simulink model "intes_cross_2018b_0110_2"  (R2018b)
settings: Solver=VariableStepAuto  StartTime=0.0  StopTime=10.0  RelTol=1e-3
values from neighbouring files (symbols this model uses):
  k_ZOP_V2X_Enable = 1.0    [ZOP_Func.sldd]
settings Model: Creator=lenovo  LastModifiedBy=lenovo

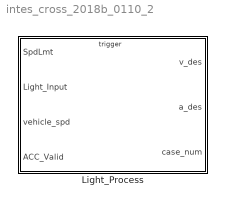
== system intes_cross_2018b_0110_2 ==
  Light_Process : Subsystem

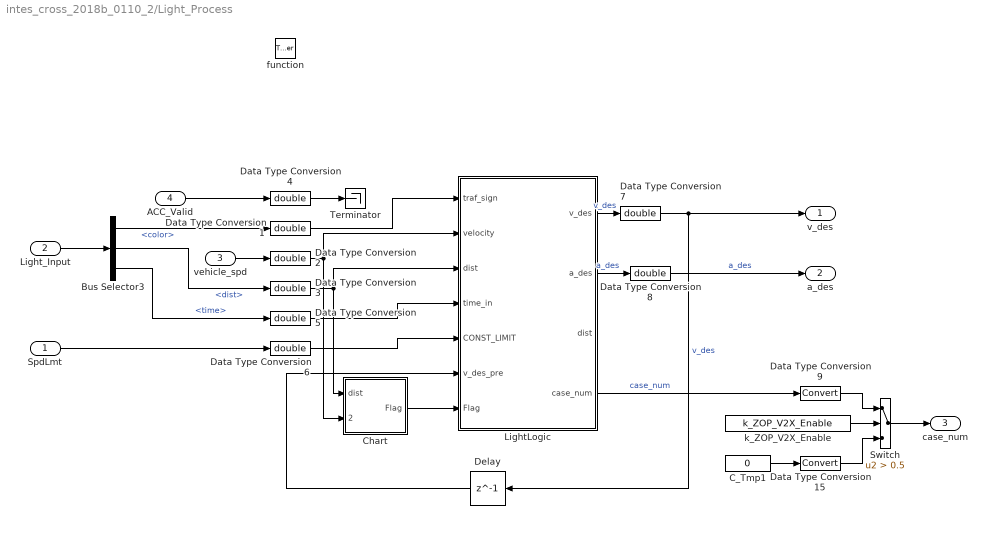
== system intes_cross_2018b_0110_2/Light_Process ==
  SpdLmt : Inport  BusOutputAsStruct=on
  Light_Input : Inport  Port=2  OutDataTypeStr=Bus: Light_Info_ST  BusOutputAsStruct=on
  vehicle_spd : Inport  Port=3  BusOutputAsStruct=on
  ACC_Valid : Inport  Port=4  BusOutputAsStruct=on
  function : TriggerPort  TriggerType=function-call  VariantControl=Variant
  Bus Selector3 : BusSelector  OutputSignals=color,dist,time
  C_Tmp1 : Constant  Value=0
  Chart : Stateflow chart  TreatAsAtomicUnit=on
  Data Type Conversion{1..8} (8 alike) : DataTypeConversion  OutDataTypeStr=double
  Data Type Conversion15 : DataTypeConversion
  Data Type Conversion9 : DataTypeConversion
  Delay : Delay  DelayLength=1
  LightLogic : MATLAB Function  TreatAsAtomicUnit=on
  Switch : Switch  Criteria=u2 > Threshold  Threshold=0.5
  Terminator : Terminator
  k_ZOP_V2X_Enable : Constant  Value=k_ZOP_V2X_Enable
  v_des : Outport
  a_des : Outport  Port=2
  case_num : Outport  Port=3
  wires:
  Data Type Conversion7/1 -> v_des/1, Delay/1  "v_des"
  Delay/1 -> LightLogic/6(v_des_pre)
  Light_Input/1 -> Bus Selector3/1
  ACC_Valid/1 -> Data Type Conversion4/1
  Data Type Conversion8/1 -> a_des/1  "a_des"
  Bus Selector3/1 -> Data Type Conversion1/1  "<color>"
  Bus Selector3/2 -> Data Type Conversion3/1  "<dist>"
  vehicle_spd/1 -> Data Type Conversion2/1
  Bus Selector3/3 -> Data Type Conversion5/1  "<time>"
  Data Type Conversion1/1 -> LightLogic/1(traf_sign)
  Data Type Conversion3/1 -> LightLogic/3("dist "), Chart/1(dist)
  Data Type Conversion5/1 -> LightLogic/4(time_in)
  Data Type Conversion6/1 -> LightLogic/5(CONST_LIMIT)
  Data Type Conversion2/1 -> LightLogic/2(velocity), Chart/2(velocity)
  SpdLmt/1 -> Data Type Conversion6/1
  LightLogic/2(a_des) -> Data Type Conversion8/1  "a_des"
  LightLogic/4(case_num) -> Data Type Conversion9/1  "case_num"
  k_ZOP_V2X_Enable/1 -> Switch/2
  C_Tmp1/1 -> Data Type Conversion15/1
  Switch/1 -> case_num/1
  Data Type Conversion15/1 -> Switch/3
  Data Type Conversion9/1 -> Switch/1
  Chart/1(Flag) -> LightLogic/7(Flag)
  LightLogic/1(v_des) -> Data Type Conversion7/1  "v_des"
  Data Type Conversion4/1 -> Terminator/1

== stateflow chart intes_cross_2018b_0110_2/Light_Process/Chart ==
  state init
    en:
    Flag=0;
  state Off
    en:
    Flag=0;
  state On
    du:
    Flag=1;
  (default) -> init
  init -> On : [dist > 0 && dist / (velocity + 0.0001) <= 5]
  Off -> init : [dist > 0]
  On -> Off : [dist < -5]
  data: dist input; velocity input; Flag output

== matlab function intes_cross_2018b_0110_2/Light_Process/LightLogic ==
  data: v_des output; a_des output; traf_sign input; velocity input; dist input; time_in input; CONST_LIMIT input; dist output; v_des_pre input; case_num output; Flag input
function [v_des,a_des,dist,case_num] = intesec_cross( traf_sign, velocity, dist, time_in,CONST_LIMIT,v_des_pre,Flag)  
%% this is a function that provide desired velocity, and distance to traffic light;
    % input: trafic_sign with green = 0; red = 1; yellow = 2;
    %        velocity in unit of kph;
    %        dist, and time is distance(m) to cross, and traffic time left
    %        CONST_LIMIT is velocity limit at cross, which is a reference CONSTANT velocity from
    %        ACC module.
    %        v_des_pre preseve previous v_des for next step use.
    
    % output: desired velocity for ACC module, in unit of kph;
    %         dist is distance(m) to front cross;
   
    case_num = 0;
    time = time_in;
    green = 1;
    red = 3;
    yellow = 2;
%     if time == 2
%         a_des = 0;
%          v_des = 0;
%     end
    
    if (Flag == 0)
        v_des = 100;
        a_des = 0;
        dist = 100;
        case_num = 0;
        return;
    end
    
    if dist < 0
        if traf_sign == green
            dist = 200;
        else
            dist = 0;
        end
    end
    
   
    
    
    if (Flag == 1)

        v = velocity;
        % CONST_LIMIT = CONST_LIMIT;
        delta_t = 0.5;

        if traf_sign == green
            time = time+3;
        elseif traf_sign == yellow
            traf_sign = green;
        end

        switch traf_sign
            case green
                
                T = time;
                a = 2 * (dist - v * T) / (T^2 + 0.0001);
                v_temp = v + a * T;

                if (a >= 1) || ((a >= 0) && (a < 1) && (v_temp >= CONST_LIMIT))
                    v_des = 0;
                    a_des = 0;
                    case_num = 1;

                elseif ((a < 0) && (v_temp >= 0) && (v_temp <= CONST_LIMIT))
                    v_des = CONST_LIMIT;
                    a_des = 0;
                    case_num = 2;
                else
                    v_des = CONST_LIMIT;
                    a_des = a;
                    case_num = 3;
                end

%                 else %(ACC_MODE == 1)
%                     T_ACC = dist / (v + 0.0001);
%                     if T_ACC < time - delta_t
%                         v_des = v;
%                         a_des = 0;
%                         case_num = 4;
% 
%                     elseif T_ACC > time + delta_t
%                         v_des = 0;
%                         a_des = 0;
%                         case_num = 5;
% 
%                     else
%                         v_des = v_des_pre;
%                         a_des = 0;
%                         case_num = 6;
%                     end
               

            case red
                
                    if (dist < 4) && (v < 1)
                        a_des = 0.25 * dist - 1;
                        v_des = 0;
                        case_num = 12;
                    else
                        T = time + 1;
                        a = 2 * (dist - v * T) / T^2;
                        v_temp = v + a * T;

                        if (a < -1)
                            v_des = 0;
                            a_des = -1;
                            case_num = 7;

                        elseif (a <=0 && a>= -1)
                            v_des = max(0,v_temp);
                            a_des = a;
                            case_num = 8;

                        elseif (a > 0 && a <= 1 && v_temp < CONST_LIMIT)
                            v_des = max(0,v_temp);
                            a_des = a;
                            case_num = 9;

                        else
                            v_des = CONST_LIMIT;
                            a_des = 0;
                            case_num = 10;

                        end
                    end
               

            otherwise
                v_des = CONST_LIMIT;
                a_des = 0;
                case_num = 11;
        end
        
    else
        v_des = 100;
        a_des = 100;
        dist = 100;
        case_num = 0;
         
    end
end
